simulink model "canonical_observable_form"  (R2021b)
settings: Solver=VariableStepAuto  StartTime=0.0  StopTime=10.0  RelTol=1e-3
settings Model: Creator=den  LastModifiedBy=den

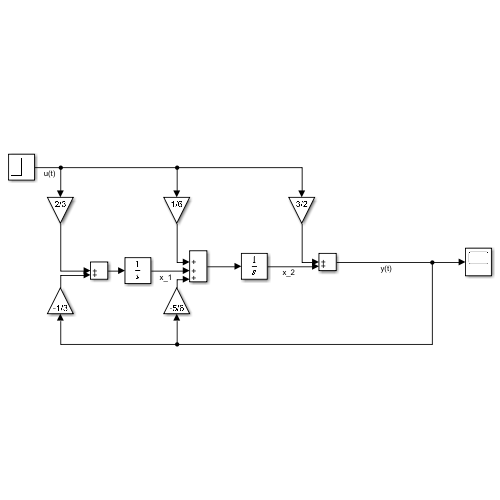
[thumbnail: Simulink's stored preview of the top-level diagram]
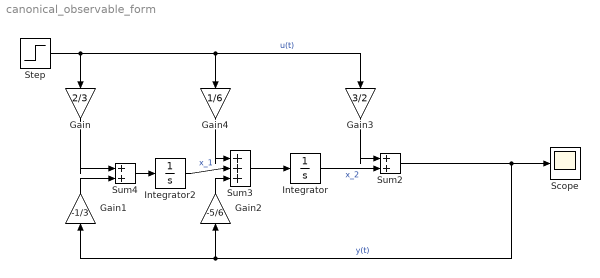
== system canonical_observable_form ==
  Gain : Gain  Gain=2/3
  Gain1 : Gain  Gain=-1/3
  Gain2 : Gain  Gain=-5/6
  Gain3 : Gain  Gain=3/2
  Gain4 : Gain  Gain=1/6
  Integrator : Integrator
  Integrator2 : Integrator
  Scope : Scope
  Step : Step  Time=0  SampleTime=0
  Sum2 : Sum  Inputs=|++
  Sum3 : Sum  Inputs=|+++
  Sum4 : Sum  Inputs=|++
  wires:
  Gain3/1 -> Sum2/1
  Sum2/1 -> Scope/1, Gain1/1, Gain2/1  "y(t)"
  Sum3/1 -> Integrator/1
  Integrator/1 -> Sum2/2  "x_2"
  Gain/1 -> Sum4/1
  Gain1/1 -> Sum4/2
  Sum4/1 -> Integrator2/1
  Gain2/1 -> Sum3/3
  Integrator2/1 -> Sum3/2  "x_1"
  Step/1 -> Gain3/1, Gain4/1, Gain/1  "u(t)"
  Gain4/1 -> Sum3/1
